simulink model "traj_track_1d"  (R2020a)
settings: Solver=VariableStepAuto  StartTime=0.0  StopTime=4  RelTol=1e-3
values from neighbouring files (symbols this model uses):
  Kg = 1    [example1D.m]
  Kp = 1    [example1D.m]
  Kv = 10    [example1D.m]
  pol_position = [ -1/3 2 0 0 ]    [example1D.m]
  pol_velocity = [ -1 4 0]    [example1D.m]
  y0 = [ -1 ; 0]    [example1D.m]
libraries: simulink x1
settings Model: Creator=Thomas  LastModifiedBy=thomas
settings SFSimCC: CustomCodeUndefinedFunction=UseInterfaceOnly

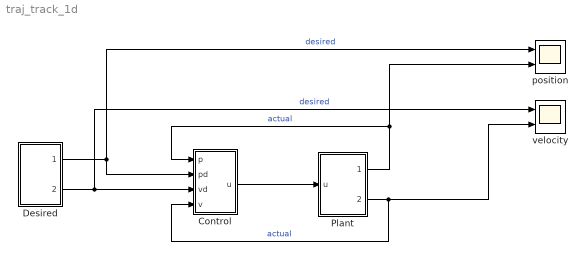
== system traj_track_1d ==
  Control : Subsystem
  Desired : Subsystem
  Plant : Subsystem
  position : Scope  NumInputPorts=2
  velocity : Scope  NumInputPorts=2
  wires:
  Desired/1(Position) -> Control/2(pd), position/1  "desired"
  Desired/2(Speed) -> Control/3(vd), velocity/1  "desired"
  Control/1(u) -> Plant/1(u)
  Plant/2(speed) -> velocity/2, Control/4(v)  "actual"
  Plant/1(position) -> position/2, Control/1(p)  "actual"

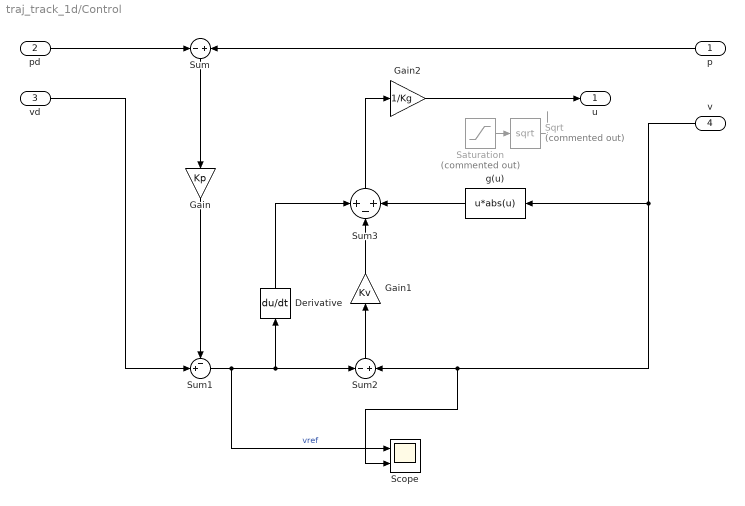
== system traj_track_1d/Control ==
  p : Inport
  pd : Inport  Port=2
  vd : Inport  Port=3
  v : Inport  Port=4
  Derivative : Derivative
  Gain : Gain  Gain=Kp
  Gain1 : Gain  Gain=Kv
  Gain2 : Gain  Gain=1/Kg
  Saturation : Saturate  Commented=on  UpperLimit=Inf  LowerLimit=0
  Scope : Scope  NumInputPorts=2
  Sqrt : Sqrt  Commented=on  SaturateOnIntegerOverflow=on
  Sum : Sum  Inputs=-+
  Sum1 : Sum  Inputs=-+|
  Sum2 : Sum  Inputs=-|+
  Sum3 : Sum  Inputs=+-+
  g(u) : Fcn  Expr=u*abs(u)
  u : Outport  VectorParamsAs1DForOutWhenUnconnected=off
  wires:
  Sum3/1 -> Gain2/1
  Sum1/1 -> Scope/1, Sum2/1, Derivative/1  "vref"
  g(u)/1 -> Sum3/3
  Gain1/1 -> Sum3/2
  Gain/1 -> Sum1/1
  v/1 -> Scope/2, Sum2/2, g(u)/1
  Derivative/1 -> Sum3/1
  Sum2/1 -> Gain1/1
  Sum/1 -> Gain/1
  p/1 -> Sum/2
  pd/1 -> Sum/1
  vd/1 -> Sum1/2
  Gain2/1 -> u/1
  Saturation/1 -> Sqrt/1
  Sqrt/1 -> ?
  ? -> Saturation/1

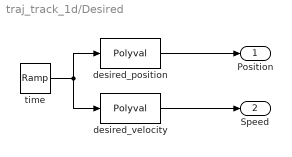
== system traj_track_1d/Desired ==
  desired_position : Polyval  Coefs=pol_position
  desired_velocity : Polyval  Coefs=pol_velocity
  time : simulink/Sources/Ramp  slope=1  start=0  InitialOutput=0
  Position : Outport  VectorParamsAs1DForOutWhenUnconnected=off
  Speed : Outport  Port=2  VectorParamsAs1DForOutWhenUnconnected=off
  wires:
  time/1 -> desired_velocity/1, desired_position/1
  desired_position/1 -> Position/1
  desired_velocity/1 -> Speed/1

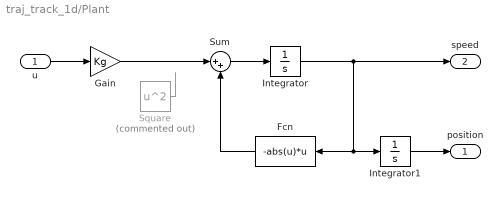
== system traj_track_1d/Plant ==
  u : Inport
  Fcn : Fcn  Expr=-abs(u)*u
  Gain : Gain  Gain=Kg
  Integrator : Integrator  InitialCondition=y0(2)
  Integrator1 : Integrator  InitialCondition=y0(1)
  Square : Math  Commented=on  Operator=square  SignedPower=on  RndMeth=Zero  SaturateOnIntegerOverflow=on
  Sum : Sum  Inputs=|++
  position : Outport  VectorParamsAs1DForOutWhenUnconnected=off
  speed : Outport  Port=2  VectorParamsAs1DForOutWhenUnconnected=off
  wires:
  Fcn/1 -> Sum/2
  Sum/1 -> Integrator/1
  Gain/1 -> Sum/1
  u/1 -> Gain/1
  Integrator1/1 -> position/1
  Integrator/1 -> speed/1, Integrator1/1, Fcn/1
  ? -> Square/1
  Square/1 -> ?
